simulink model "EMC_no_gaze"  (R2015a)
settings: Solver=ode4  SolverMode=MultiTasking  StartTime=0.0  StopTime=inf  FixedStep=BKIN_STEP_TIME  RelTol=1e-3
StartFcn:
  |  warndlg('Dexterit-E models cannot run under simulation. Please compile your model and run it from within Dexterit-E.');set_param(bdroot,'SimulationCommand','stop')
model workspace (MAT data in the model file):
  BKIN_KINEMATIC_FRAME_SIZE = 400
  BKIN_STEP_TIME = 0.00025
  COLOR = 4
  COL_X = 1
  COL_Y = 2
  E_NO_EVENT = 0
  LOAD_X = 1
  LOAD_Y = 2
  MOVEMENT_DELAY = 3
  PATH_LENGTH = 1
  PATH_PERIOD = 2
  POST_TRIAL_DELAY = 4
  RADIUS = 3
  TRAJECTORY = 1
  TRAJECTORY_TYPE = 2
  TRIAL_END = 3
  TRIAL_MOVEMENT = 2
  TRIAL_RESET = 4
  TRIAL_START = 1
  X_POSITION = 1
  Y_POSITION = 2
  col_x = 1
  col_y = 2
  ANGULAR_THRESHOLD = 5
  GAZE_EXIT = 6
  START_REACHED = 7
  FIXATION_DURATION = 6
  TRACKING_TARGET_ROW = 7
  FEEDBACK_COLOR = 5
  CROSS_LOGICAL_RADIUS = 8
  DETECT_FIXATION = 8
  GAZE_IN_TARGET = 5
  START_STABILIZATION = 9
  HAND_IN_TARGET = 9
  BACKGROUND_LOAD = 10
  DIST_BETWEEN_TRAJ = 11
libraries: simulink x14, xpcrtudplib x12, xpcutilitieslib x10, xpcobsoletelib x8, ethercat x2, General x2, Video x2, KINARM_EP_loads x1, KINARM_general x1
(part 7 of 7)

== matlab function EMC_no_gaze/DataLogging/apply loads/verify NaN ==
  data: torques_in input; torques_out output
function torques_out  = fcn(torques_in)
%#codegen

persistent check isWorking

if isempty(check)
    check = 1;

    % The code generator tries to be very smart when converting this to C.
    % if you do something simple like isinf(inf) or isnan(nan) then those
    % statements are optimized out of the C for always being true. The code
    % below is an attempt to outsmart the converted to actually generate
    % real C code that should generate nan or inf. From what I can tell,
    % at least in R2018a this gets generated to proper code that does these
    % checks the way I want.
    
    sq = rand();
    while sq > 0.99
        sq = rand();
    end
    
    r = ceil(rand());
    mr = -r;
    r = r * 2;
    
    % DEX-3729, DEX-3732
    % if the wrong compiler options are used then "fast math" could be
    % enabled. Fast math breaks checks for NaN. If we can't tell if a number
    % is NaN then we need to force all output forces to zero.
    % it appears that checking for inf always works, but checking for
    % isfinite is broken with isnan.
    if ~isnan(sqrt(sq - 0.99)) || ~isinf(1.0 / (r + mr + mr))
        isWorking = 0;
        fprintf('***WARNING****');
        fprintf('Checks for NaN/inf FAIL. No forces will be produced.\n')
    else
        isWorking = 1;
        fprintf('Checks for NaN/inf WORK.\n')
    end
    
end

torques_out = torques_in;

% DEX-3729, DEX-3732
% if the wrong compiler options are used then "fast math" could be
% enabled. Fast math breaks checks for NaN. If we can't tell if a number
% is NaN then we need to force all output forces to zero.
if isWorking
    if sum(isnan(torques_out)) > 0
        torques_out(isnan(torques_out)) = 0;
    end
    
    if sum(isinf(torques_out)) > 0
        torques_out(isinf(torques_out)) = 0;
    end
else
    torques_out(:) = 0;
end

== matlab function EMC_no_gaze/DataLogging/compare encoders/delta ==
  data: secondaryEncAngles input; deltas output; primaryEncAngles input
function deltas = fcn(secondaryEncAngles, primaryEncAngles)
%#eml

deltas = secondaryEncAngles - primaryEncAngles;

== matlab function EMC_no_gaze/DataLogging/create_lab_info/Subsystem/MATLAB Function ==
  data: orientation input; is_right_arm output; has_secondary input; isEP input; isExo output; has_high_res_encoders output
function [is_right_arm, isExo, has_high_res_encoders] = fcn(orientation, has_secondary, isEP)
%#codegen

isExo = 1;
if isEP
    isExo = 0;
end

has_high_res_encoders = has_secondary;

is_right_arm = 0;
if (isExo && orientation == 1) || (isEP && orientation == -1)
    is_right_arm = 1;
end

== matlab function EMC_no_gaze/DataLogging/create_lab_info/Subsystem/MATLAB Function1 ==
  data: orientation input; is_right_arm output; has_secondary input; isEP input; isExo output; has_high_res_encoders output
function [is_right_arm, isExo, has_high_res_encoders] = fcn(orientation, has_secondary, isEP)
%#codegen

isExo = 1;
if isEP
    isExo = 0;
end

has_high_res_encoders = has_secondary;

is_right_arm = 0;
if (isExo && orientation == 1) || (isEP && orientation == -1)
    is_right_arm = 1;
end

== matlab function EMC_no_gaze/DataLogging/monitor torques/MATLAB Function ==
  data: robot_failures output; torque_err_bitfield output; cmd input; abs_diff output; rec input; threshold_rel_diff input; rel_diff output; threshold_abs_diff input
function [robot_failures, torque_err_bitfield, abs_diff, rel_diff] = fcn(cmd, rec, threshold_rel_diff, threshold_abs_diff)
%#codegen

abs_diff = abs(cmd - rec);
rel_diff = abs_diff ./ cmd;
rel_diff(~isfinite(rel_diff)) = 0;

out_of_spec_motors = (abs_diff >= threshold_abs_diff) + (rel_diff >= threshold_rel_diff);
robot_failures = [sum(out_of_spec_motors(1:2) == 2) > 0, sum(out_of_spec_motors(3:4) == 2) > 0];
torque_errors = out_of_spec_motors == 2;
torque_err_bitfield = sum(bitshift(uint32(torque_errors'), 0:3));

== stateflow chart EMC_no_gaze/DataLogging/monitor torques/torque_monitor ==
  state init/
    command_multiplier = 1;
    stop_vel_mode = 0;
    robot_err_bits_out = 0;
  state Done/
  state Monitoring/
  state EpMonitor/
    state Robot1/ [parallel]
      settings: executionOrder=1
      state not_holding/
      state Waiting/
      note: After the current limit stops we need
          | to wait a bit before currents are back to full force
      state CurrentLimited/
      state Pause/
      state Err/
        command_multiplier = 0;
        stop_vel_mode = 1;
      (default) -> EpMonitor.Robot1.Waiting
      EpMonitor.Robot1.Waiting -> EpMonitor.Robot1.not_holding [order 1] : [e_grips[1] == 0 || robot_scaling[1] != 1]
      EpMonitor.Robot1.not_holding -> EpMonitor.Robot1.Waiting : [e_grips[1] == 1 && robot_scaling[1] == 1]
      EpMonitor.Robot1.Waiting -> (junction 47) [order 2]
      EpMonitor.Robot1.Pause -> EpMonitor.Robot1.not_holding : after(1000, e_clk)
      EpMonitor.Robot1.CurrentLimited -> EpMonitor.Robot1.Pause : [current_limit_enabled[1] == 0]
      (junction 47) -> EpMonitor.Robot1.CurrentLimited [order 1] : [current_limit_enabled[1] != 0]
      (junction 47) -> EpMonitor.Robot1.Err [order 2] : [robot_error[1] == 1]
          | {robot_err_bits_out = robot_err_bits_in;}
    state Robot2/ [parallel]
      settings: executionOrder=2
      state not_holding/
      state Waiting/
      state CurrentLimited/
      state Pause/
      state Err/
        command_multiplier = 0;
        stop_vel_mode = 1;
      (default) -> EpMonitor.Robot2.Waiting
      EpMonitor.Robot2.Waiting -> EpMonitor.Robot2.not_holding [order 1] : [e_grips[2] == 0 || robot_scaling[2] != 1]
      EpMonitor.Robot2.not_holding -> EpMonitor.Robot2.Waiting : [e_grips[2] == 1 && robot_scaling[2] == 1]
      EpMonitor.Robot2.Waiting -> (junction 68) [order 2]
      EpMonitor.Robot2.Pause -> EpMonitor.Robot2.not_holding : after(1000, e_clk)
      EpMonitor.Robot2.CurrentLimited -> EpMonitor.Robot2.Pause : [current_limit_enabled[2] == 0]
      (junction 68) -> EpMonitor.Robot2.CurrentLimited [order 1] : [current_limit_enabled[2] != 0]
      (junction 68) -> EpMonitor.Robot2.Err [order 2] : [robot_error[2] == 1]
          | {robot_err_bits_out = robot_err_bits_in;}
  state ExoMonitor/
  state eStopdown/
  state Wait/
  state CurrentLimited/
  state ErrorFound/
    command_multiplier = 0;
  (default) -> init
  init -> Done [order 1] : [is_ecat == 0]
  init -> Monitoring [order 2] : after(2000, e_clk)
  Monitoring -> EpMonitor [order 1] : [is_ep == 1]
  Monitoring -> ExoMonitor [order 2]
  ExoMonitor -> eStopdown [order 1] : [robot_scaling[1] != 1 || robot_scaling[2] != 1]
  eStopdown -> ExoMonitor : [robot_scaling[1] == 1 && robot_scaling[2] == 1]
  Wait -> eStopdown : after(1000, e_clk)
  ExoMonitor -> (junction 80) [order 2]
  (junction 84) -> Wait
  CurrentLimited -> (junction 84) : [current_limit_enabled[3] == 0]
  (junction 80) -> CurrentLimited [order 2] : [current_limit_enabled[3] != 0]
  (junction 80) -> ErrorFound [order 1] : [robot_error[1] == 1 || robot_error[2] == 1]
      | {robot_err_bits_out = robot_err_bits_in;}
  data: e_grips input size=2; robot_scaling input double size=2; current_limit_enabled input double size=3; command_multiplier output double size=1; is_ep input double; is_ecat input boolean; robot_error input size=2; stop_vel_mode output double; robot_err_bits_in input double; robot_err_bits_out output double
  events: e_clk input RISING_EDGE_EVENT
